simulink model "Final_EWASP_VC"  (R2022a)
settings: Solver=ode1  StartTime=0.0  StopTime=24*3600  FixedStep=10  RelTol=1e-3
values from neighbouring files (symbols this model uses):
  Aux_Threshold = 52    [Setup_Code_EWASP_VC.m]
  buildingAge = 2005    [Setup_Code_EWASP_VC.m]
  ceilingHeight = 2.4    [Setup_Code_EWASP_VC.m]
  conductiveHconnectMatrix = [ ... (first row only)    [Setup_Code_EWASP_VC.m]
  cRoofGreen = 100000    [Setup_Code_EWASP_VC.m]
  Defrost_After_Time = 30    [Setup_Code_EWASP_VC.m]
  DHWDemandProfile = occFreegainHotwaterElecTestPassiveOcc3(:,3)    [Setup_Code_EWASP_VC.m]
  Elec_Max = Elec_Max*(30/24.2)    [Setup_Code_EWASP_VC.m]
  Elec_Mid = Elec_Mid*(30/24.2)    [Setup_Code_EWASP_VC.m]
  Elec_Min = Elec_Min*(30/24.2)    [Setup_Code_EWASP_VC.m]
  ElecDemandProfile = occFreegainHotwaterElecTestPassiveOcc3(:,4)    [Setup_Code_EWASP_VC.m]
  ElecFixed = [Elec_Max(6,2) Elec_Max(6,4) Elec_Max(6,6) Elec_Max(6,7) ... (first row only)    [Setup_Code_EWASP_VC.m]
  floorOrCeilingArea = floorOrCeilingArea*1.15    [Setup_Code_EWASP_VC.m]
  forceCold = 0    [Setup_Code_EWASP_VC.m]
  freegain = occFreegainHotwaterElecTestPassiveOcc3(:,2)-max(occupancy)*25    [Setup_Code_EWASP_VC.m]
  furnitureModelOn = 1    [Setup_Code_EWASP_VC.m]
  Heat_Max = Heat_Max*(30/24.2)    [Setup_Code_EWASP_VC.m]
  Heat_Mid = Heat_Mid*(30/24.2)    [Setup_Code_EWASP_VC.m]
  Heat_Min = Heat_Min*(30/24.2)    [Setup_Code_EWASP_VC.m]
  HeatFixed = [Heat_Max(6,2) Heat_Max(6,4) Heat_Max(6,6) Heat_Max(6,7) ... (first row only)    [Setup_Code_EWASP_VC.m]
  HeatingOnProfile = repmat(HeatingOnProfile,365,1)    [Setup_Code_EWASP_VC.m]
  HEX_ReturnLowerLimit = 52.5    [Setup_Code_EWASP_VC.m]
  HEX_ReturnUpperLimit = 55    [Setup_Code_EWASP_VC.m]
  LeakMultiplier = 1+(2*(rand()-0.5)/10)    [Setup_Code_EWASP_VC.m]
  loopCap = 15    [Setup_Code_EWASP_VC.m]
  maxOcc = max(occupancyProfile)    [Setup_Code_EWASP_VC.m]
  NESW_wallArea = max(NESW_Lengths*ceilingHeight-NESW_Windows,0)    [Setup_Code_EWASP_VC.m]
  NESW_Windows = [ ... (first row only)    [Setup_Code_EWASP_VC.m]
  numRooms = roomCount    [Setup_Code_EWASP_VC.m]
  offsetDays = 0    [Setup_Code_EWASP_VC.m]
  pumpChoice = pumpChoices(MinIndex,1)    [Setup_Code_EWASP_VC.m]
  pumpRamp = 180    [Setup_Code_EWASP_VC.m]
  ReturnLowerLimit = 37.5    [Setup_Code_EWASP_VC.m]
  ReturnUpperLimit = 40    [Setup_Code_EWASP_VC.m]
  RoofIrradiance = Flat_NS_EW_RoofIrradiance(:,1)    [Setup_Code_EWASP_VC.m]
  roofStartTemp = ones(11,1)*20    [Setup_Code_EWASP_VC.m]
  rooftype = 0    [Setup_Code_EWASP_VC.m]
  RoomDataMatrix = [zeros(1,12);ones(1,12)*wallDensity;zeros(1,12);ones(1,12)*wallU;ones(1,12)*windowU;ones(1,12)*floorU;ones(1,12)*ceilingU;zeros(1,12);windowArea, 0;floorOrCeilingArea;zeros(1,12);floorOrCeilingArea*ceilingHeight]    [Setup_Code_EWASP_VC.m]
  roomVol = roomVol*1.15    [Setup_Code_EWASP_VC.m]
  slabStartTemp = (GroundTempTimeSeries(offsetDays*1440+1,1)+thermostatSetting)/2    [Setup_Code_EWASP_VC.m]
  SlackRequest = zeros(1440,1)    [Setup_Code_EWASP_VC.m]
  SolarThermalExists = 0    [Setup_Code_EWASP_VC.m]
  SourceFixed = HeatFixed-ElecFixed    [Setup_Code_EWASP_VC.m]
  StateSeries = StateSeriesGenerator(22,7,1)    [Setup_Code_EWASP_VC.m]
  Tank_Lower_Temp = 49.5    [Setup_Code_EWASP_VC.m]
  Tank_Upper_Temp = 52    [Setup_Code_EWASP_VC.m]
  Tank_Volume_m3 = 0.15    [Setup_Code_EWASP_VC.m]
  TankHeatHour = randi([1 5])-1    [Setup_Code_EWASP_VC.m]
  thermostatSetting = 20.0    (= 20)    [Setup_Code_EWASP_VC.m]
  upDown = [0;0;0;0;1;1;1;1;1;1;1]    [Setup_Code_EWASP_VC.m]
  variableASHP = 1    [Setup_Code_EWASP_VC.m]
  wallStartTempExt = thermostatSetting*(0.266+0.00215*outdoorStartTemp+0.018*wallU+0.00113*outdoorStartTemp*wallU+0.0068*wallU^2)    [Setup_Code_EWASP_VC.m]
undefined symbols (not defined in the file or in its folder): a, ceilingU, condUDMatrix, convUDMatrix, deltaPEXPANDED_E, deltaPEXPANDED_E2, deltaPEXPANDED_N, deltaPEXPANDED_N2, deltaPEXPANDED_S, deltaPEXPANDED_S2, deltaPEXPANDED_W, deltaPEXPANDED_W2, DesiredDHWTemp, DesiredFlowTempVsInOutDeltaTemp, DiffuseHorizontal, DiscIntNeverNeededParam, DNI, dwnAndConcrete, DWORK_A_HX, DWORK_CHK_FLU, DWORK_CP_NODE, DWORK_DH, DWORK_FLUID, DWORK_HCON, DWORK_LOSS, DWORK_MDOTDOWN, DWORK_MDOTIN, DWORK_MDOTUP, DWORK_MIX, DWORK_PRESS, DWORK_QDOTIN, DWORK_RHO_NODE, DWORK_TIN, DWORK_TS_OLD, DWORK_V_NODE, GroundTempTimeSeries, HCM, HCM2, HCM_closed, HCM_closed2, intermediateU, IsTop, massFlowMatrix, neighbourMatrix, numericalRoomUse, RadiatorMatrix, room2roomflowmatrix_E, room2roomflowmatrix_E2, room2roomflowmatrix_N, room2roomflowmatrix_N2, room2roomflowmatrix_S, room2roomflowmatrix_S2, room2roomflowmatrix_W, room2roomflowmatrix_W2, StateAirInEXPANDED_E, StateAirInEXPANDED_E2, StateAirInEXPANDED_N, StateAirInEXPANDED_N2, StateAirInEXPANDED_S, StateAirInEXPANDED_S2 ... (+23)
libraries: simulink x6, dspsigops x4, dspmtrx3 x4, carnot x3, spsEdgeDetectorLib x2, dspstat3 x2, powerlib_meascontrol x1, simulink_extras x1
(part 25 of 27)

== matlab function Final_EWASP_VC/Subsystem_Room2/Kitchen/furniture/MATLAB Function ==
  data: roomArea input; woodPlasticHeatTransfertoroom output; roomtype input; roomTemp input; TemperatureWoodPlastic input; TemperatureSoft input; deltaTWoodPlasticMean output; softHeatTransfertoroom output; deltaTsoftMean output
function [woodPlasticHeatTransfertoroom,deltaTWoodPlasticMean,softHeatTransfertoroom,deltaTsoftMean]=FurnitureTransfer(roomArea,roomtype,roomTemp,TemperatureWoodPlastic,TemperatureSoft)

excessMeanWoodPlastic=TemperatureWoodPlastic-roomTemp;
excessMeanSoft=TemperatureSoft-roomTemp;

if roomtype==1
    
%carpetMass=roomArea*2.041;% 2.041kg/m2 based on  https://thecarpetstop.co.uk/buying-guides/#:~:text=These%20are%20given%20in%20ounces,commonly%20a%20more%20luxurious%20carpet.  
%underlayMass=roomArea*2.7;% 2.7kg/m2 based on https://www.carpet-underlay-shop.co.uk/products/duralay-durafit-650-15-07m2-from-5-74-per-m2
CurtainMass=15;
Sofafabricmass=10;% based on 2lb/ft^3 and 2 sofas - 3 seater and 2 seater https://furnitureblog.simplicitysofas.com/blog/what-is-the-difference-between-a-sofa-cushions-foam-density-and-firmness/ 
matressMass=0; %no beds
duvetandSheetsMass=0; %no beds

SoftMass=CurtainMass+Sofafabricmass;
woodPlasticMass=roomArea*20-SoftMass;

elseif roomtype ==2

%carpetMass=roomArea*2.041;% 2.041kg/m2 based on  https://thecarpetstop.co.uk/buying-guides/#:~:text=These%20are%20given%20in%20ounces,commonly%20a%20more%20luxurious%20carpet.  
%underlayMass=roomArea*2.7;% 2.7kg/m2 based on https://www.carpet-underlay-shop.co.uk/products/duralay-durafit-650-15-07m2-from-5-74-per-m2
CurtainMass=15;
matressMass=40; %https://democracy.york.gov.uk/documents/s2116/Annex%20C%20REcycling%20Report%20frnweights2005.pdf
duvetandSheetsMass=5; %5kg based on %https://inthewash.co.uk/washing-machines/can-you-wash-a-king-size-duvet-in-an-8-9-10-kg-washing-machine/#:~:text=A%20king%20size%20duvet%20will,able%20to%20cope%20with%20them.
Sofafabricmass=0; %no sofa

SoftMass=CurtainMass+matressMass+duvetandSheetsMass;


woodPlasticMass=roomArea*30-SoftMass;
woodPlasticMass=roomArea*30-SoftMass;

else %room is other e.g. kitchen - assume heavily furnished, and majority wood or plastic
    
CurtainMass=0; %
matressMass=0; %
duvetandSheetsMass=0; %
Sofafabricmass=0; %no sofa

SoftMass=0;

woodPlasticMass=roomArea*35-SoftMass;
woodPlasticMass=roomArea*35-SoftMass;    
    
end





softDensityA=60;
softDensityB=80;
softThicknessA=0.15; %represents thicker furnishings (sofa foam etc.)
softThicknessB=0.01; %Represents thinner funishings (e.g. carpet)

SoftMassA=duvetandSheetsMass+Sofafabricmass+matressMass;
SoftMassB=CurtainMass;

SoftVolumeA=SoftMassA/softDensityA;
SoftVolumeB=SoftMassA/softDensityB;

approxSoftA_SA=(SoftVolumeA/softThicknessA);%no 2* here due to one surface usually being obscured
approxSoftB_SA=(SoftVolumeB/softThicknessB);%as above

Softradius=3*((SoftVolumeA+SoftVolumeB)/(approxSoftA_SA+approxSoftB_SA));
SoftbiotNumber=(10/0.03)*((SoftVolumeA+SoftVolumeB)/(approxSoftA_SA+approxSoftB_SA));% appropriate for typical soft furnishings with conductivity 0.03 w/mK and convective transfer coefficient 10 W/k m2 
SoftFBI=1/(0.282*SoftbiotNumber+0.944);
excessSurfSoft=SoftFBI*excessMeanSoft;
softHeatTransfertoroom=excessSurfSoft*10*(approxSoftA_SA+approxSoftB_SA);
deltaTsoftMean=-softHeatTransfertoroom/(softDensityA*SoftVolumeA*1400+softDensityB*SoftVolumeB*1400);

if isnan(deltaTsoftMean)==1
deltaTsoftMean=0;
else
end
    
woodPlasticDensity=800; %600kg/m^3 as of Influence of internal thermal mass on the indoor thermal dynamics and integration of phase change materials in furniture for building energy storage: A review
woodPlasticThickness=0.018; %0.018m typical as of as of Influence of internal thermal mass on the indoor thermal dynamics and integration of phase change materials in furniture for building energy storage: A review
woodPlasticVolume=woodPlasticMass/woodPlasticDensity;
approxWoodPlasticSA=(woodPlasticVolume/woodPlasticThickness); %a rough surface area calculation for the wooden elements

radius=3*woodPlasticVolume/approxWoodPlasticSA;
biotNumber=(10/0.2)*(woodPlasticVolume/approxWoodPlasticSA);% appropriate for typical wood with conductivity 0.2 w/mK and convective transfer coefficient 10 W/k m2 
FBI=1/(0.282*biotNumber+0.944);
excessSurfWoodPlastic=FBI*excessMeanWoodPlastic;
woodPlasticHeatTransfertoroom=excessSurfWoodPlastic*10*approxWoodPlasticSA;
deltaTWoodPlasticMean=-woodPlasticHeatTransfertoroom/(800*woodPlasticVolume*1700);% heat capacity of wodd and plastic is assumer 1700 J/Kg, they are very close in capacity anyway (1.76 wood, 1.67 plastic)

deltaTWoodPlasticMean(isnan(deltaTWoodPlasticMean))=0;

softHeatTransfertoroom(isnan(softHeatTransfertoroom))=0;

%end

== matlab function Final_EWASP_VC/Subsystem_Room3/Utility/furniture/MATLAB Function ==
  data: roomArea input; woodPlasticHeatTransfertoroom output; roomtype input; roomTemp input; TemperatureWoodPlastic input; TemperatureSoft input; deltaTWoodPlasticMean output; softHeatTransfertoroom output; deltaTsoftMean output
function [woodPlasticHeatTransfertoroom,deltaTWoodPlasticMean,softHeatTransfertoroom,deltaTsoftMean]=FurnitureTransfer(roomArea,roomtype,roomTemp,TemperatureWoodPlastic,TemperatureSoft)

excessMeanWoodPlastic=TemperatureWoodPlastic-roomTemp;
excessMeanSoft=TemperatureSoft-roomTemp;

if roomtype==1
    
%carpetMass=roomArea*2.041;% 2.041kg/m2 based on  https://thecarpetstop.co.uk/buying-guides/#:~:text=These%20are%20given%20in%20ounces,commonly%20a%20more%20luxurious%20carpet.  
%underlayMass=roomArea*2.7;% 2.7kg/m2 based on https://www.carpet-underlay-shop.co.uk/products/duralay-durafit-650-15-07m2-from-5-74-per-m2
CurtainMass=15;
Sofafabricmass=10;% based on 2lb/ft^3 and 2 sofas - 3 seater and 2 seater https://furnitureblog.simplicitysofas.com/blog/what-is-the-difference-between-a-sofa-cushions-foam-density-and-firmness/ 
matressMass=0; %no beds
duvetandSheetsMass=0; %no beds

SoftMass=CurtainMass+Sofafabricmass;
woodPlasticMass=roomArea*20-SoftMass;

elseif roomtype ==2

%carpetMass=roomArea*2.041;% 2.041kg/m2 based on  https://thecarpetstop.co.uk/buying-guides/#:~:text=These%20are%20given%20in%20ounces,commonly%20a%20more%20luxurious%20carpet.  
%underlayMass=roomArea*2.7;% 2.7kg/m2 based on https://www.carpet-underlay-shop.co.uk/products/duralay-durafit-650-15-07m2-from-5-74-per-m2
CurtainMass=15;
matressMass=40; %https://democracy.york.gov.uk/documents/s2116/Annex%20C%20REcycling%20Report%20frnweights2005.pdf
duvetandSheetsMass=5; %5kg based on %https://inthewash.co.uk/washing-machines/can-you-wash-a-king-size-duvet-in-an-8-9-10-kg-washing-machine/#:~:text=A%20king%20size%20duvet%20will,able%20to%20cope%20with%20them.
Sofafabricmass=0; %no sofa

SoftMass=CurtainMass+matressMass+duvetandSheetsMass;


woodPlasticMass=roomArea*30-SoftMass;
woodPlasticMass=roomArea*30-SoftMass;

else %room is other e.g. kitchen - assume heavily furnished, and majority wood or plastic
    
CurtainMass=0; %
matressMass=0; %
duvetandSheetsMass=0; %
Sofafabricmass=0; %no sofa

SoftMass=0;

woodPlasticMass=roomArea*35-SoftMass;
woodPlasticMass=roomArea*35-SoftMass;    
    
end





softDensityA=60;
softDensityB=80;
softThicknessA=0.15; %represents thicker furnishings (sofa foam etc.)
softThicknessB=0.01; %Represents thinner funishings (e.g. carpet)

SoftMassA=duvetandSheetsMass+Sofafabricmass+matressMass;
SoftMassB=CurtainMass;

SoftVolumeA=SoftMassA/softDensityA;
SoftVolumeB=SoftMassA/softDensityB;

approxSoftA_SA=(SoftVolumeA/softThicknessA);%no 2* here due to one surface usually being obscured
approxSoftB_SA=(SoftVolumeB/softThicknessB);%as above

Softradius=3*((SoftVolumeA+SoftVolumeB)/(approxSoftA_SA+approxSoftB_SA));
SoftbiotNumber=(10/0.03)*((SoftVolumeA+SoftVolumeB)/(approxSoftA_SA+approxSoftB_SA));% appropriate for typical soft furnishings with conductivity 0.03 w/mK and convective transfer coefficient 10 W/k m2 
SoftFBI=1/(0.282*SoftbiotNumber+0.944);
excessSurfSoft=SoftFBI*excessMeanSoft;
softHeatTransfertoroom=excessSurfSoft*10*(approxSoftA_SA+approxSoftB_SA);
deltaTsoftMean=-softHeatTransfertoroom/(softDensityA*SoftVolumeA*1400+softDensityB*SoftVolumeB*1400);

if isnan(deltaTsoftMean)==1
deltaTsoftMean=0;
else
end
    
woodPlasticDensity=800; %600kg/m^3 as of Influence of internal thermal mass on the indoor thermal dynamics and integration of phase change materials in furniture for building energy storage: A review
woodPlasticThickness=0.018; %0.018m typical as of as of Influence of internal thermal mass on the indoor thermal dynamics and integration of phase change materials in furniture for building energy storage: A review
woodPlasticVolume=woodPlasticMass/woodPlasticDensity;
approxWoodPlasticSA=(woodPlasticVolume/woodPlasticThickness); %a rough surface area calculation for the wooden elements

radius=3*woodPlasticVolume/approxWoodPlasticSA;
biotNumber=(10/0.2)*(woodPlasticVolume/approxWoodPlasticSA);% appropriate for typical wood with conductivity 0.2 w/mK and convective transfer coefficient 10 W/k m2 
FBI=1/(0.282*biotNumber+0.944);
excessSurfWoodPlastic=FBI*excessMeanWoodPlastic;
woodPlasticHeatTransfertoroom=excessSurfWoodPlastic*10*approxWoodPlasticSA;
deltaTWoodPlasticMean=-woodPlasticHeatTransfertoroom/(800*woodPlasticVolume*1700);% heat capacity of wodd and plastic is assumer 1700 J/Kg, they are very close in capacity anyway (1.76 wood, 1.67 plastic)

deltaTWoodPlasticMean(isnan(deltaTWoodPlasticMean))=0;

softHeatTransfertoroom(isnan(softHeatTransfertoroom))=0;

%end

== matlab function Final_EWASP_VC/Subsystem_Room4/Hall/furniture/MATLAB Function ==
  data: roomArea input; woodPlasticHeatTransfertoroom output; roomtype input; roomTemp input; TemperatureWoodPlastic input; TemperatureSoft input; deltaTWoodPlasticMean output; softHeatTransfertoroom output; deltaTsoftMean output
function [woodPlasticHeatTransfertoroom,deltaTWoodPlasticMean,softHeatTransfertoroom,deltaTsoftMean]=FurnitureTransfer(roomArea,roomtype,roomTemp,TemperatureWoodPlastic,TemperatureSoft)

excessMeanWoodPlastic=TemperatureWoodPlastic-roomTemp;
excessMeanSoft=TemperatureSoft-roomTemp;

if roomtype==1
    
%carpetMass=roomArea*2.041;% 2.041kg/m2 based on  https://thecarpetstop.co.uk/buying-guides/#:~:text=These%20are%20given%20in%20ounces,commonly%20a%20more%20luxurious%20carpet.  
%underlayMass=roomArea*2.7;% 2.7kg/m2 based on https://www.carpet-underlay-shop.co.uk/products/duralay-durafit-650-15-07m2-from-5-74-per-m2
CurtainMass=15;
Sofafabricmass=10;% based on 2lb/ft^3 and 2 sofas - 3 seater and 2 seater https://furnitureblog.simplicitysofas.com/blog/what-is-the-difference-between-a-sofa-cushions-foam-density-and-firmness/ 
matressMass=0; %no beds
duvetandSheetsMass=0; %no beds

SoftMass=CurtainMass+Sofafabricmass;
woodPlasticMass=roomArea*20-SoftMass;

elseif roomtype ==2

%carpetMass=roomArea*2.041;% 2.041kg/m2 based on  https://thecarpetstop.co.uk/buying-guides/#:~:text=These%20are%20given%20in%20ounces,commonly%20a%20more%20luxurious%20carpet.  
%underlayMass=roomArea*2.7;% 2.7kg/m2 based on https://www.carpet-underlay-shop.co.uk/products/duralay-durafit-650-15-07m2-from-5-74-per-m2
CurtainMass=15;
matressMass=40; %https://democracy.york.gov.uk/documents/s2116/Annex%20C%20REcycling%20Report%20frnweights2005.pdf
duvetandSheetsMass=5; %5kg based on %https://inthewash.co.uk/washing-machines/can-you-wash-a-king-size-duvet-in-an-8-9-10-kg-washing-machine/#:~:text=A%20king%20size%20duvet%20will,able%20to%20cope%20with%20them.
Sofafabricmass=0; %no sofa

SoftMass=CurtainMass+matressMass+duvetandSheetsMass;


woodPlasticMass=roomArea*30-SoftMass;
woodPlasticMass=roomArea*30-SoftMass;

else %room is other e.g. kitchen - assume heavily furnished, and majority wood or plastic
    
CurtainMass=0; %
matressMass=0; %
duvetandSheetsMass=0; %
Sofafabricmass=0; %no sofa

SoftMass=0;

woodPlasticMass=roomArea*35-SoftMass;
woodPlasticMass=roomArea*35-SoftMass;    
    
end





softDensityA=60;
softDensityB=80;
softThicknessA=0.15; %represents thicker furnishings (sofa foam etc.)
softThicknessB=0.01; %Represents thinner funishings (e.g. carpet)

SoftMassA=duvetandSheetsMass+Sofafabricmass+matressMass;
SoftMassB=CurtainMass;

SoftVolumeA=SoftMassA/softDensityA;
SoftVolumeB=SoftMassA/softDensityB;

approxSoftA_SA=(SoftVolumeA/softThicknessA);%no 2* here due to one surface usually being obscured
approxSoftB_SA=(SoftVolumeB/softThicknessB);%as above

Softradius=3*((SoftVolumeA+SoftVolumeB)/(approxSoftA_SA+approxSoftB_SA));
SoftbiotNumber=(10/0.03)*((SoftVolumeA+SoftVolumeB)/(approxSoftA_SA+approxSoftB_SA));% appropriate for typical soft furnishings with conductivity 0.03 w/mK and convective transfer coefficient 10 W/k m2 
SoftFBI=1/(0.282*SoftbiotNumber+0.944);
excessSurfSoft=SoftFBI*excessMeanSoft;
softHeatTransfertoroom=excessSurfSoft*10*(approxSoftA_SA+approxSoftB_SA);
deltaTsoftMean=-softHeatTransfertoroom/(softDensityA*SoftVolumeA*1400+softDensityB*SoftVolumeB*1400);

if isnan(deltaTsoftMean)==1
deltaTsoftMean=0;
else
end
    
woodPlasticDensity=800; %600kg/m^3 as of Influence of internal thermal mass on the indoor thermal dynamics and integration of phase change materials in furniture for building energy storage: A review
woodPlasticThickness=0.018; %0.018m typical as of as of Influence of internal thermal mass on the indoor thermal dynamics and integration of phase change materials in furniture for building energy storage: A review
woodPlasticVolume=woodPlasticMass/woodPlasticDensity;
approxWoodPlasticSA=(woodPlasticVolume/woodPlasticThickness); %a rough surface area calculation for the wooden elements

radius=3*woodPlasticVolume/approxWoodPlasticSA;
biotNumber=(10/0.2)*(woodPlasticVolume/approxWoodPlasticSA);% appropriate for typical wood with conductivity 0.2 w/mK and convective transfer coefficient 10 W/k m2 
FBI=1/(0.282*biotNumber+0.944);
excessSurfWoodPlastic=FBI*excessMeanWoodPlastic;
woodPlasticHeatTransfertoroom=excessSurfWoodPlastic*10*approxWoodPlasticSA;
deltaTWoodPlasticMean=-woodPlasticHeatTransfertoroom/(800*woodPlasticVolume*1700);% heat capacity of wodd and plastic is assumer 1700 J/Kg, they are very close in capacity anyway (1.76 wood, 1.67 plastic)

deltaTWoodPlasticMean(isnan(deltaTWoodPlasticMean))=0;

softHeatTransfertoroom(isnan(softHeatTransfertoroom))=0;

%end

== matlab function Final_EWASP_VC/Subsystem_Room5/Landing/furniture/MATLAB Function ==
  data: roomArea input; woodPlasticHeatTransfertoroom output; roomtype input; roomTemp input; TemperatureWoodPlastic input; TemperatureSoft input; deltaTWoodPlasticMean output; softHeatTransfertoroom output; deltaTsoftMean output
function [woodPlasticHeatTransfertoroom,deltaTWoodPlasticMean,softHeatTransfertoroom,deltaTsoftMean]=FurnitureTransfer(roomArea,roomtype,roomTemp,TemperatureWoodPlastic,TemperatureSoft)

excessMeanWoodPlastic=TemperatureWoodPlastic-roomTemp;
excessMeanSoft=TemperatureSoft-roomTemp;

if roomtype==1
    
%carpetMass=roomArea*2.041;% 2.041kg/m2 based on  https://thecarpetstop.co.uk/buying-guides/#:~:text=These%20are%20given%20in%20ounces,commonly%20a%20more%20luxurious%20carpet.  
%underlayMass=roomArea*2.7;% 2.7kg/m2 based on https://www.carpet-underlay-shop.co.uk/products/duralay-durafit-650-15-07m2-from-5-74-per-m2
CurtainMass=15;
Sofafabricmass=10;% based on 2lb/ft^3 and 2 sofas - 3 seater and 2 seater https://furnitureblog.simplicitysofas.com/blog/what-is-the-difference-between-a-sofa-cushions-foam-density-and-firmness/ 
matressMass=0; %no beds
duvetandSheetsMass=0; %no beds

SoftMass=CurtainMass+Sofafabricmass;
woodPlasticMass=roomArea*20-SoftMass;

elseif roomtype ==2

%carpetMass=roomArea*2.041;% 2.041kg/m2 based on  https://thecarpetstop.co.uk/buying-guides/#:~:text=These%20are%20given%20in%20ounces,commonly%20a%20more%20luxurious%20carpet.  
%underlayMass=roomArea*2.7;% 2.7kg/m2 based on https://www.carpet-underlay-shop.co.uk/products/duralay-durafit-650-15-07m2-from-5-74-per-m2
CurtainMass=15;
matressMass=40; %https://democracy.york.gov.uk/documents/s2116/Annex%20C%20REcycling%20Report%20frnweights2005.pdf
duvetandSheetsMass=5; %5kg based on %https://inthewash.co.uk/washing-machines/can-you-wash-a-king-size-duvet-in-an-8-9-10-kg-washing-machine/#:~:text=A%20king%20size%20duvet%20will,able%20to%20cope%20with%20them.
Sofafabricmass=0; %no sofa

SoftMass=CurtainMass+matressMass+duvetandSheetsMass;


woodPlasticMass=roomArea*30-SoftMass;
woodPlasticMass=roomArea*30-SoftMass;

else %room is other e.g. kitchen - assume heavily furnished, and majority wood or plastic
    
CurtainMass=0; %
matressMass=0; %
duvetandSheetsMass=0; %
Sofafabricmass=0; %no sofa

SoftMass=0;

woodPlasticMass=roomArea*35-SoftMass;
woodPlasticMass=roomArea*35-SoftMass;    
    
end





softDensityA=60;
softDensityB=80;
softThicknessA=0.15; %represents thicker furnishings (sofa foam etc.)
softThicknessB=0.01; %Represents thinner funishings (e.g. carpet)

SoftMassA=duvetandSheetsMass+Sofafabricmass+matressMass;
SoftMassB=CurtainMass;

SoftVolumeA=SoftMassA/softDensityA;
SoftVolumeB=SoftMassA/softDensityB;

approxSoftA_SA=(SoftVolumeA/softThicknessA);%no 2* here due to one surface usually being obscured
approxSoftB_SA=(SoftVolumeB/softThicknessB);%as above

Softradius=3*((SoftVolumeA+SoftVolumeB)/(approxSoftA_SA+approxSoftB_SA));
SoftbiotNumber=(10/0.03)*((SoftVolumeA+SoftVolumeB)/(approxSoftA_SA+approxSoftB_SA));% appropriate for typical soft furnishings with conductivity 0.03 w/mK and convective transfer coefficient 10 W/k m2 
SoftFBI=1/(0.282*SoftbiotNumber+0.944);
excessSurfSoft=SoftFBI*excessMeanSoft;
softHeatTransfertoroom=excessSurfSoft*10*(approxSoftA_SA+approxSoftB_SA);
deltaTsoftMean=-softHeatTransfertoroom/(softDensityA*SoftVolumeA*1400+softDensityB*SoftVolumeB*1400);

if isnan(deltaTsoftMean)==1
deltaTsoftMean=0;
else
end
    
woodPlasticDensity=800; %600kg/m^3 as of Influence of internal thermal mass on the indoor thermal dynamics and integration of phase change materials in furniture for building energy storage: A review
woodPlasticThickness=0.018; %0.018m typical as of as of Influence of internal thermal mass on the indoor thermal dynamics and integration of phase change materials in furniture for building energy storage: A review
woodPlasticVolume=woodPlasticMass/woodPlasticDensity;
approxWoodPlasticSA=(woodPlasticVolume/woodPlasticThickness); %a rough surface area calculation for the wooden elements

radius=3*woodPlasticVolume/approxWoodPlasticSA;
biotNumber=(10/0.2)*(woodPlasticVolume/approxWoodPlasticSA);% appropriate for typical wood with conductivity 0.2 w/mK and convective transfer coefficient 10 W/k m2 
FBI=1/(0.282*biotNumber+0.944);
excessSurfWoodPlastic=FBI*excessMeanWoodPlastic;
woodPlasticHeatTransfertoroom=excessSurfWoodPlastic*10*approxWoodPlasticSA;
deltaTWoodPlasticMean=-woodPlasticHeatTransfertoroom/(800*woodPlasticVolume*1700);% heat capacity of wodd and plastic is assumer 1700 J/Kg, they are very close in capacity anyway (1.76 wood, 1.67 plastic)

deltaTWoodPlasticMean(isnan(deltaTWoodPlasticMean))=0;

softHeatTransfertoroom(isnan(softHeatTransfertoroom))=0;

%end

== matlab function Final_EWASP_VC/Subsystem_Room4/Hall/Subsystem1/MATLAB Function1 ==
  data: PU_AreaIrradianceTotal output; angleSeries input; NEWS_Irradiance output; DNISeries input; DiffSeries input; Time input; offsetDays input; SurfaceAlbedo input; NESW_wallArea input; roomNumber input; c_OutPU input; deltaTexternalNEWS output
function [PU_AreaIrradianceTotal, NEWS_Irradiance,deltaTexternalNEWS] = SolarSeriesToExtWallGains(angleSeries,DNISeries,DiffSeries,Time,offsetDays,SurfaceAlbedo,NESW_wallArea,roomNumber,c_OutPU)

%deltaTexternalNEWS=zeros(1,4);

Angle_NEWS=angleSeries(ceil((offsetDays*1440)+Time/60+0.00001),1:4);
DNI=DNISeries(ceil((offsetDays*1440)+Time/60+0.00001),1);

PU_AreaDiff=DiffSeries(ceil((offsetDays*1440)+Time/60+0.00001),1)/2;%extracts correct Diff for the timestep, factor of 1/2 corrects for 90 degree walls (so only half Diff irradiance can be utilised)
PU_AreaDNI=cos(deg2rad(Angle_NEWS))*DNI;
NEWS_wallArea=NESW_wallArea;
NEWS_wallArea([3 4],:)=NEWS_wallArea([4 3],:);

RoomWallAreas_NEWS=NEWS_wallArea(:,roomNumber)';
PU_AreaIrradianceTotal=(PU_AreaDNI+PU_AreaDiff)*(1-SurfaceAlbedo);

NEWS_Irradiance=RoomWallAreas_NEWS.*PU_AreaIrradianceTotal;
deltaTexternalNEWS=NEWS_Irradiance./(c_OutPU*RoomWallAreas_NEWS);

for i=1:4
   
    if RoomWallAreas_NEWS(1,i)==0
        deltaTexternalNEWS(1,i)=0;
    else
        
    end
    
end

== matlab function Final_EWASP_VC/Subsystem_Room6/Bedroom1/furniture/MATLAB Function ==
  data: roomArea input; woodPlasticHeatTransfertoroom output; roomtype input; roomTemp input; TemperatureWoodPlastic input; TemperatureSoft input; deltaTWoodPlasticMean output; softHeatTransfertoroom output; deltaTsoftMean output
function [woodPlasticHeatTransfertoroom,deltaTWoodPlasticMean,softHeatTransfertoroom,deltaTsoftMean]=FurnitureTransfer(roomArea,roomtype,roomTemp,TemperatureWoodPlastic,TemperatureSoft)

excessMeanWoodPlastic=TemperatureWoodPlastic-roomTemp;
excessMeanSoft=TemperatureSoft-roomTemp;

if roomtype==1
    
%carpetMass=roomArea*2.041;% 2.041kg/m2 based on  https://thecarpetstop.co.uk/buying-guides/#:~:text=These%20are%20given%20in%20ounces,commonly%20a%20more%20luxurious%20carpet.  
%underlayMass=roomArea*2.7;% 2.7kg/m2 based on https://www.carpet-underlay-shop.co.uk/products/duralay-durafit-650-15-07m2-from-5-74-per-m2
CurtainMass=15;
Sofafabricmass=10;% based on 2lb/ft^3 and 2 sofas - 3 seater and 2 seater https://furnitureblog.simplicitysofas.com/blog/what-is-the-difference-between-a-sofa-cushions-foam-density-and-firmness/ 
matressMass=0; %no beds
duvetandSheetsMass=0; %no beds

SoftMass=CurtainMass+Sofafabricmass;
woodPlasticMass=roomArea*20-SoftMass;

elseif roomtype ==2

%carpetMass=roomArea*2.041;% 2.041kg/m2 based on  https://thecarpetstop.co.uk/buying-guides/#:~:text=These%20are%20given%20in%20ounces,commonly%20a%20more%20luxurious%20carpet.  
%underlayMass=roomArea*2.7;% 2.7kg/m2 based on https://www.carpet-underlay-shop.co.uk/products/duralay-durafit-650-15-07m2-from-5-74-per-m2
CurtainMass=15;
matressMass=40; %https://democracy.york.gov.uk/documents/s2116/Annex%20C%20REcycling%20Report%20frnweights2005.pdf
duvetandSheetsMass=5; %5kg based on %https://inthewash.co.uk/washing-machines/can-you-wash-a-king-size-duvet-in-an-8-9-10-kg-washing-machine/#:~:text=A%20king%20size%20duvet%20will,able%20to%20cope%20with%20them.
Sofafabricmass=0; %no sofa

SoftMass=CurtainMass+matressMass+duvetandSheetsMass;


woodPlasticMass=roomArea*30-SoftMass;
woodPlasticMass=roomArea*30-SoftMass;

else %room is other e.g. kitchen - assume heavily furnished, and majority wood or plastic
    
CurtainMass=0; %
matressMass=0; %
duvetandSheetsMass=0; %
Sofafabricmass=0; %no sofa

SoftMass=0;

woodPlasticMass=roomArea*35-SoftMass;
woodPlasticMass=roomArea*35-SoftMass;    
    
end





softDensityA=60;
softDensityB=80;
softThicknessA=0.15; %represents thicker furnishings (sofa foam etc.)
softThicknessB=0.01; %Represents thinner funishings (e.g. carpet)

SoftMassA=duvetandSheetsMass+Sofafabricmass+matressMass;
SoftMassB=CurtainMass;

SoftVolumeA=SoftMassA/softDensityA;
SoftVolumeB=SoftMassA/softDensityB;

approxSoftA_SA=(SoftVolumeA/softThicknessA);%no 2* here due to one surface usually being obscured
approxSoftB_SA=(SoftVolumeB/softThicknessB);%as above

Softradius=3*((SoftVolumeA+SoftVolumeB)/(approxSoftA_SA+approxSoftB_SA));
SoftbiotNumber=(10/0.03)*((SoftVolumeA+SoftVolumeB)/(approxSoftA_SA+approxSoftB_SA));% appropriate for typical soft furnishings with conductivity 0.03 w/mK and convective transfer coefficient 10 W/k m2 
SoftFBI=1/(0.282*SoftbiotNumber+0.944);
excessSurfSoft=SoftFBI*excessMeanSoft;
softHeatTransfertoroom=excessSurfSoft*10*(approxSoftA_SA+approxSoftB_SA);
deltaTsoftMean=-softHeatTransfertoroom/(softDensityA*SoftVolumeA*1400+softDensityB*SoftVolumeB*1400);

if isnan(deltaTsoftMean)==1
deltaTsoftMean=0;
else
end
    
woodPlasticDensity=800; %600kg/m^3 as of Influence of internal thermal mass on the indoor thermal dynamics and integration of phase change materials in furniture for building energy storage: A review
woodPlasticThickness=0.018; %0.018m typical as of as of Influence of internal thermal mass on the indoor thermal dynamics and integration of phase change materials in furniture for building energy storage: A review
woodPlasticVolume=woodPlasticMass/woodPlasticDensity;
approxWoodPlasticSA=(woodPlasticVolume/woodPlasticThickness); %a rough surface area calculation for the wooden elements

radius=3*woodPlasticVolume/approxWoodPlasticSA;
biotNumber=(10/0.2)*(woodPlasticVolume/approxWoodPlasticSA);% appropriate for typical wood with conductivity 0.2 w/mK and convective transfer coefficient 10 W/k m2 
FBI=1/(0.282*biotNumber+0.944);
excessSurfWoodPlastic=FBI*excessMeanWoodPlastic;
woodPlasticHeatTransfertoroom=excessSurfWoodPlastic*10*approxWoodPlasticSA;
deltaTWoodPlasticMean=-woodPlasticHeatTransfertoroom/(800*woodPlasticVolume*1700);% heat capacity of wodd and plastic is assumer 1700 J/Kg, they are very close in capacity anyway (1.76 wood, 1.67 plastic)

deltaTWoodPlasticMean(isnan(deltaTWoodPlasticMean))=0;

softHeatTransfertoroom(isnan(softHeatTransfertoroom))=0;

%end

== matlab function Final_EWASP_VC/Subsystem_Room7/Bedroom 2/furniture/MATLAB Function ==
  data: roomArea input; woodPlasticHeatTransfertoroom output; roomtype input; roomTemp input; TemperatureWoodPlastic input; TemperatureSoft input; deltaTWoodPlasticMean output; softHeatTransfertoroom output; deltaTsoftMean output
function [woodPlasticHeatTransfertoroom,deltaTWoodPlasticMean,softHeatTransfertoroom,deltaTsoftMean]=FurnitureTransfer(roomArea,roomtype,roomTemp,TemperatureWoodPlastic,TemperatureSoft)

excessMeanWoodPlastic=TemperatureWoodPlastic-roomTemp;
excessMeanSoft=TemperatureSoft-roomTemp;

if roomtype==1
    
%carpetMass=roomArea*2.041;% 2.041kg/m2 based on  https://thecarpetstop.co.uk/buying-guides/#:~:text=These%20are%20given%20in%20ounces,commonly%20a%20more%20luxurious%20carpet.  
%underlayMass=roomArea*2.7;% 2.7kg/m2 based on https://www.carpet-underlay-shop.co.uk/products/duralay-durafit-650-15-07m2-from-5-74-per-m2
CurtainMass=15;
Sofafabricmass=10;% based on 2lb/ft^3 and 2 sofas - 3 seater and 2 seater https://furnitureblog.simplicitysofas.com/blog/what-is-the-difference-between-a-sofa-cushions-foam-density-and-firmness/ 
matressMass=0; %no beds
duvetandSheetsMass=0; %no beds

SoftMass=CurtainMass+Sofafabricmass;
woodPlasticMass=roomArea*20-SoftMass;

elseif roomtype ==2

%carpetMass=roomArea*2.041;% 2.041kg/m2 based on  https://thecarpetstop.co.uk/buying-guides/#:~:text=These%20are%20given%20in%20ounces,commonly%20a%20more%20luxurious%20carpet.  
%underlayMass=roomArea*2.7;% 2.7kg/m2 based on https://www.carpet-underlay-shop.co.uk/products/duralay-durafit-650-15-07m2-from-5-74-per-m2
CurtainMass=15;
matressMass=40; %https://democracy.york.gov.uk/documents/s2116/Annex%20C%20REcycling%20Report%20frnweights2005.pdf
duvetandSheetsMass=5; %5kg based on %https://inthewash.co.uk/washing-machines/can-you-wash-a-king-size-duvet-in-an-8-9-10-kg-washing-machine/#:~:text=A%20king%20size%20duvet%20will,able%20to%20cope%20with%20them.
Sofafabricmass=0; %no sofa

SoftMass=CurtainMass+matressMass+duvetandSheetsMass;


woodPlasticMass=roomArea*30-SoftMass;
woodPlasticMass=roomArea*30-SoftMass;

else %room is other e.g. kitchen - assume heavily furnished, and majority wood or plastic
    
CurtainMass=0; %
matressMass=0; %
duvetandSheetsMass=0; %
Sofafabricmass=0; %no sofa

SoftMass=0;

woodPlasticMass=roomArea*35-SoftMass;
woodPlasticMass=roomArea*35-SoftMass;    
    
end





softDensityA=60;
softDensityB=80;
softThicknessA=0.15; %represents thicker furnishings (sofa foam etc.)
softThicknessB=0.01; %Represents thinner funishings (e.g. carpet)

SoftMassA=duvetandSheetsMass+Sofafabricmass+matressMass;
SoftMassB=CurtainMass;

SoftVolumeA=SoftMassA/softDensityA;
SoftVolumeB=SoftMassA/softDensityB;

approxSoftA_SA=(SoftVolumeA/softThicknessA);%no 2* here due to one surface usually being obscured
approxSoftB_SA=(SoftVolumeB/softThicknessB);%as above

Softradius=3*((SoftVolumeA+SoftVolumeB)/(approxSoftA_SA+approxSoftB_SA));
SoftbiotNumber=(10/0.03)*((SoftVolumeA+SoftVolumeB)/(approxSoftA_SA+approxSoftB_SA));% appropriate for typical soft furnishings with conductivity 0.03 w/mK and convective transfer coefficient 10 W/k m2 
SoftFBI=1/(0.282*SoftbiotNumber+0.944);
excessSurfSoft=SoftFBI*excessMeanSoft;
softHeatTransfertoroom=excessSurfSoft*10*(approxSoftA_SA+approxSoftB_SA);
deltaTsoftMean=-softHeatTransfertoroom/(softDensityA*SoftVolumeA*1400+softDensityB*SoftVolumeB*1400);

if isnan(deltaTsoftMean)==1
deltaTsoftMean=0;
else
end
    
woodPlasticDensity=800; %600kg/m^3 as of Influence of internal thermal mass on the indoor thermal dynamics and integration of phase change materials in furniture for building energy storage: A review
woodPlasticThickness=0.018; %0.018m typical as of as of Influence of internal thermal mass on the indoor thermal dynamics and integration of phase change materials in furniture for building energy storage: A review
woodPlasticVolume=woodPlasticMass/woodPlasticDensity;
approxWoodPlasticSA=(woodPlasticVolume/woodPlasticThickness); %a rough surface area calculation for the wooden elements

radius=3*woodPlasticVolume/approxWoodPlasticSA;
biotNumber=(10/0.2)*(woodPlasticVolume/approxWoodPlasticSA);% appropriate for typical wood with conductivity 0.2 w/mK and convective transfer coefficient 10 W/k m2 
FBI=1/(0.282*biotNumber+0.944);
excessSurfWoodPlastic=FBI*excessMeanWoodPlastic;
woodPlasticHeatTransfertoroom=excessSurfWoodPlastic*10*approxWoodPlasticSA;
deltaTWoodPlasticMean=-woodPlasticHeatTransfertoroom/(800*woodPlasticVolume*1700);% heat capacity of wodd and plastic is assumer 1700 J/Kg, they are very close in capacity anyway (1.76 wood, 1.67 plastic)

deltaTWoodPlasticMean(isnan(deltaTWoodPlasticMean))=0;

softHeatTransfertoroom(isnan(softHeatTransfertoroom))=0;

%end

== matlab function Final_EWASP_VC/Subsystem_Room8/Bedroom3/furniture/MATLAB Function ==
  data: roomArea input; woodPlasticHeatTransfertoroom output; roomtype input; roomTemp input; TemperatureWoodPlastic input; TemperatureSoft input; deltaTWoodPlasticMean output; softHeatTransfertoroom output; deltaTsoftMean output
function [woodPlasticHeatTransfertoroom,deltaTWoodPlasticMean,softHeatTransfertoroom,deltaTsoftMean]=FurnitureTransfer(roomArea,roomtype,roomTemp,TemperatureWoodPlastic,TemperatureSoft)

excessMeanWoodPlastic=TemperatureWoodPlastic-roomTemp;
excessMeanSoft=TemperatureSoft-roomTemp;

if roomtype==1
    
%carpetMass=roomArea*2.041;% 2.041kg/m2 based on  https://thecarpetstop.co.uk/buying-guides/#:~:text=These%20are%20given%20in%20ounces,commonly%20a%20more%20luxurious%20carpet.  
%underlayMass=roomArea*2.7;% 2.7kg/m2 based on https://www.carpet-underlay-shop.co.uk/products/duralay-durafit-650-15-07m2-from-5-74-per-m2
CurtainMass=15;
Sofafabricmass=10;% based on 2lb/ft^3 and 2 sofas - 3 seater and 2 seater https://furnitureblog.simplicitysofas.com/blog/what-is-the-difference-between-a-sofa-cushions-foam-density-and-firmness/ 
matressMass=0; %no beds
duvetandSheetsMass=0; %no beds

SoftMass=CurtainMass+Sofafabricmass;
woodPlasticMass=roomArea*20-SoftMass;

elseif roomtype ==2

%carpetMass=roomArea*2.041;% 2.041kg/m2 based on  https://thecarpetstop.co.uk/buying-guides/#:~:text=These%20are%20given%20in%20ounces,commonly%20a%20more%20luxurious%20carpet.  
%underlayMass=roomArea*2.7;% 2.7kg/m2 based on https://www.carpet-underlay-shop.co.uk/products/duralay-durafit-650-15-07m2-from-5-74-per-m2
CurtainMass=15;
matressMass=40; %https://democracy.york.gov.uk/documents/s2116/Annex%20C%20REcycling%20Report%20frnweights2005.pdf
duvetandSheetsMass=5; %5kg based on %https://inthewash.co.uk/washing-machines/can-you-wash-a-king-size-duvet-in-an-8-9-10-kg-washing-machine/#:~:text=A%20king%20size%20duvet%20will,able%20to%20cope%20with%20them.
Sofafabricmass=0; %no sofa

SoftMass=CurtainMass+matressMass+duvetandSheetsMass;


woodPlasticMass=roomArea*30-SoftMass;
woodPlasticMass=roomArea*30-SoftMass;

else %room is other e.g. kitchen - assume heavily furnished, and majority wood or plastic
    
CurtainMass=0; %
matressMass=0; %
duvetandSheetsMass=0; %
Sofafabricmass=0; %no sofa

SoftMass=0;

woodPlasticMass=roomArea*35-SoftMass;
woodPlasticMass=roomArea*35-SoftMass;    
    
end





softDensityA=60;
softDensityB=80;
softThicknessA=0.15; %represents thicker furnishings (sofa foam etc.)
softThicknessB=0.01; %Represents thinner funishings (e.g. carpet)

SoftMassA=duvetandSheetsMass+Sofafabricmass+matressMass;
SoftMassB=CurtainMass;

SoftVolumeA=SoftMassA/softDensityA;
SoftVolumeB=SoftMassA/softDensityB;

approxSoftA_SA=(SoftVolumeA/softThicknessA);%no 2* here due to one surface usually being obscured
approxSoftB_SA=(SoftVolumeB/softThicknessB);%as above

Softradius=3*((SoftVolumeA+SoftVolumeB)/(approxSoftA_SA+approxSoftB_SA));
SoftbiotNumber=(10/0.03)*((SoftVolumeA+SoftVolumeB)/(approxSoftA_SA+approxSoftB_SA));% appropriate for typical soft furnishings with conductivity 0.03 w/mK and convective transfer coefficient 10 W/k m2 
SoftFBI=1/(0.282*SoftbiotNumber+0.944);
excessSurfSoft=SoftFBI*excessMeanSoft;
softHeatTransfertoroom=excessSurfSoft*10*(approxSoftA_SA+approxSoftB_SA);
deltaTsoftMean=-softHeatTransfertoroom/(softDensityA*SoftVolumeA*1400+softDensityB*SoftVolumeB*1400);

if isnan(deltaTsoftMean)==1
deltaTsoftMean=0;
else
end
    
woodPlasticDensity=800; %600kg/m^3 as of Influence of internal thermal mass on the indoor thermal dynamics and integration of phase change materials in furniture for building energy storage: A review
woodPlasticThickness=0.018; %0.018m typical as of as of Influence of internal thermal mass on the indoor thermal dynamics and integration of phase change materials in furniture for building energy storage: A review
woodPlasticVolume=woodPlasticMass/woodPlasticDensity;
approxWoodPlasticSA=(woodPlasticVolume/woodPlasticThickness); %a rough surface area calculation for the wooden elements

radius=3*woodPlasticVolume/approxWoodPlasticSA;
biotNumber=(10/0.2)*(woodPlasticVolume/approxWoodPlasticSA);% appropriate for typical wood with conductivity 0.2 w/mK and convective transfer coefficient 10 W/k m2 
FBI=1/(0.282*biotNumber+0.944);
excessSurfWoodPlastic=FBI*excessMeanWoodPlastic;
woodPlasticHeatTransfertoroom=excessSurfWoodPlastic*10*approxWoodPlasticSA;
deltaTWoodPlasticMean=-woodPlasticHeatTransfertoroom/(800*woodPlasticVolume*1700);% heat capacity of wodd and plastic is assumer 1700 J/Kg, they are very close in capacity anyway (1.76 wood, 1.67 plastic)

deltaTWoodPlasticMean(isnan(deltaTWoodPlasticMean))=0;

softHeatTransfertoroom(isnan(softHeatTransfertoroom))=0;

%end

== matlab function Final_EWASP_VC/Subsystem_Room9/Bedroom4/furniture/MATLAB Function ==
  data: roomArea input; woodPlasticHeatTransfertoroom output; roomtype input; roomTemp input; TemperatureWoodPlastic input; TemperatureSoft input; deltaTWoodPlasticMean output; softHeatTransfertoroom output; deltaTsoftMean output
function [woodPlasticHeatTransfertoroom,deltaTWoodPlasticMean,softHeatTransfertoroom,deltaTsoftMean]=FurnitureTransfer(roomArea,roomtype,roomTemp,TemperatureWoodPlastic,TemperatureSoft)

excessMeanWoodPlastic=TemperatureWoodPlastic-roomTemp;
excessMeanSoft=TemperatureSoft-roomTemp;

if roomtype==1
    
%carpetMass=roomArea*2.041;% 2.041kg/m2 based on  https://thecarpetstop.co.uk/buying-guides/#:~:text=These%20are%20given%20in%20ounces,commonly%20a%20more%20luxurious%20carpet.  
%underlayMass=roomArea*2.7;% 2.7kg/m2 based on https://www.carpet-underlay-shop.co.uk/products/duralay-durafit-650-15-07m2-from-5-74-per-m2
CurtainMass=15;
Sofafabricmass=10;% based on 2lb/ft^3 and 2 sofas - 3 seater and 2 seater https://furnitureblog.simplicitysofas.com/blog/what-is-the-difference-between-a-sofa-cushions-foam-density-and-firmness/ 
matressMass=0; %no beds
duvetandSheetsMass=0; %no beds

SoftMass=CurtainMass+Sofafabricmass;
woodPlasticMass=roomArea*20-SoftMass;

elseif roomtype ==2

%carpetMass=roomArea*2.041;% 2.041kg/m2 based on  https://thecarpetstop.co.uk/buying-guides/#:~:text=These%20are%20given%20in%20ounces,commonly%20a%20more%20luxurious%20carpet.  
%underlayMass=roomArea*2.7;% 2.7kg/m2 based on https://www.carpet-underlay-shop.co.uk/products/duralay-durafit-650-15-07m2-from-5-74-per-m2
CurtainMass=15;
matressMass=40; %https://democracy.york.gov.uk/documents/s2116/Annex%20C%20REcycling%20Report%20frnweights2005.pdf
duvetandSheetsMass=5; %5kg based on %https://inthewash.co.uk/washing-machines/can-you-wash-a-king-size-duvet-in-an-8-9-10-kg-washing-machine/#:~:text=A%20king%20size%20duvet%20will,able%20to%20cope%20with%20them.
Sofafabricmass=0; %no sofa

SoftMass=CurtainMass+matressMass+duvetandSheetsMass;


woodPlasticMass=roomArea*30-SoftMass;
woodPlasticMass=roomArea*30-SoftMass;

else %room is other e.g. kitchen - assume heavily furnished, and majority wood or plastic
    
CurtainMass=0; %
matressMass=0; %
duvetandSheetsMass=0; %
Sofafabricmass=0; %no sofa

SoftMass=0;

woodPlasticMass=roomArea*35-SoftMass;
woodPlasticMass=roomArea*35-SoftMass;    
    
end





softDensityA=60;
softDensityB=80;
softThicknessA=0.15; %represents thicker furnishings (sofa foam etc.)
softThicknessB=0.01; %Represents thinner funishings (e.g. carpet)

SoftMassA=duvetandSheetsMass+Sofafabricmass+matressMass;
SoftMassB=CurtainMass;

SoftVolumeA=SoftMassA/softDensityA;
SoftVolumeB=SoftMassA/softDensityB;

approxSoftA_SA=(SoftVolumeA/softThicknessA);%no 2* here due to one surface usually being obscured
approxSoftB_SA=(SoftVolumeB/softThicknessB);%as above

Softradius=3*((SoftVolumeA+SoftVolumeB)/(approxSoftA_SA+approxSoftB_SA));
SoftbiotNumber=(10/0.03)*((SoftVolumeA+SoftVolumeB)/(approxSoftA_SA+approxSoftB_SA));% appropriate for typical soft furnishings with conductivity 0.03 w/mK and convective transfer coefficient 10 W/k m2 
SoftFBI=1/(0.282*SoftbiotNumber+0.944);
excessSurfSoft=SoftFBI*excessMeanSoft;
softHeatTransfertoroom=excessSurfSoft*10*(approxSoftA_SA+approxSoftB_SA);
deltaTsoftMean=-softHeatTransfertoroom/(softDensityA*SoftVolumeA*1400+softDensityB*SoftVolumeB*1400);

if isnan(deltaTsoftMean)==1
deltaTsoftMean=0;
else
end
    
woodPlasticDensity=800; %600kg/m^3 as of Influence of internal thermal mass on the indoor thermal dynamics and integration of phase change materials in furniture for building energy storage: A review
woodPlasticThickness=0.018; %0.018m typical as of as of Influence of internal thermal mass on the indoor thermal dynamics and integration of phase change materials in furniture for building energy storage: A review
woodPlasticVolume=woodPlasticMass/woodPlasticDensity;
approxWoodPlasticSA=(woodPlasticVolume/woodPlasticThickness); %a rough surface area calculation for the wooden elements

radius=3*woodPlasticVolume/approxWoodPlasticSA;
biotNumber=(10/0.2)*(woodPlasticVolume/approxWoodPlasticSA);% appropriate for typical wood with conductivity 0.2 w/mK and convective transfer coefficient 10 W/k m2 
FBI=1/(0.282*biotNumber+0.944);
excessSurfWoodPlastic=FBI*excessMeanWoodPlastic;
woodPlasticHeatTransfertoroom=excessSurfWoodPlastic*10*approxWoodPlasticSA;
deltaTWoodPlasticMean=-woodPlasticHeatTransfertoroom/(800*woodPlasticVolume*1700);% heat capacity of wodd and plastic is assumer 1700 J/Kg, they are very close in capacity anyway (1.76 wood, 1.67 plastic)

deltaTWoodPlasticMean(isnan(deltaTWoodPlasticMean))=0;

softHeatTransfertoroom(isnan(softHeatTransfertoroom))=0;

%end

== matlab function Final_EWASP_VC/Subsystem_Room10/En suite/furniture/MATLAB Function ==
  data: roomArea input; woodPlasticHeatTransfertoroom output; roomtype input; roomTemp input; TemperatureWoodPlastic input; TemperatureSoft input; deltaTWoodPlasticMean output; softHeatTransfertoroom output; deltaTsoftMean output
function [woodPlasticHeatTransfertoroom,deltaTWoodPlasticMean,softHeatTransfertoroom,deltaTsoftMean]=FurnitureTransfer(roomArea,roomtype,roomTemp,TemperatureWoodPlastic,TemperatureSoft)

excessMeanWoodPlastic=TemperatureWoodPlastic-roomTemp;
excessMeanSoft=TemperatureSoft-roomTemp;

if roomtype==1
    
%carpetMass=roomArea*2.041;% 2.041kg/m2 based on  https://thecarpetstop.co.uk/buying-guides/#:~:text=These%20are%20given%20in%20ounces,commonly%20a%20more%20luxurious%20carpet.  
%underlayMass=roomArea*2.7;% 2.7kg/m2 based on https://www.carpet-underlay-shop.co.uk/products/duralay-durafit-650-15-07m2-from-5-74-per-m2
CurtainMass=15;
Sofafabricmass=10;% based on 2lb/ft^3 and 2 sofas - 3 seater and 2 seater https://furnitureblog.simplicitysofas.com/blog/what-is-the-difference-between-a-sofa-cushions-foam-density-and-firmness/ 
matressMass=0; %no beds
duvetandSheetsMass=0; %no beds

SoftMass=CurtainMass+Sofafabricmass;
woodPlasticMass=roomArea*20-SoftMass;

elseif roomtype ==2

%carpetMass=roomArea*2.041;% 2.041kg/m2 based on  https://thecarpetstop.co.uk/buying-guides/#:~:text=These%20are%20given%20in%20ounces,commonly%20a%20more%20luxurious%20carpet.  
%underlayMass=roomArea*2.7;% 2.7kg/m2 based on https://www.carpet-underlay-shop.co.uk/products/duralay-durafit-650-15-07m2-from-5-74-per-m2
CurtainMass=15;
matressMass=40; %https://democracy.york.gov.uk/documents/s2116/Annex%20C%20REcycling%20Report%20frnweights2005.pdf
duvetandSheetsMass=5; %5kg based on %https://inthewash.co.uk/washing-machines/can-you-wash-a-king-size-duvet-in-an-8-9-10-kg-washing-machine/#:~:text=A%20king%20size%20duvet%20will,able%20to%20cope%20with%20them.
Sofafabricmass=0; %no sofa

SoftMass=CurtainMass+matressMass+duvetandSheetsMass;


woodPlasticMass=roomArea*30-SoftMass;
woodPlasticMass=roomArea*30-SoftMass;

else %room is other e.g. kitchen - assume heavily furnished, and majority wood or plastic
    
CurtainMass=0; %
matressMass=0; %
duvetandSheetsMass=0; %
Sofafabricmass=0; %no sofa

SoftMass=0;

woodPlasticMass=roomArea*35-SoftMass;
woodPlasticMass=roomArea*35-SoftMass;    
    
end





softDensityA=60;
softDensityB=80;
softThicknessA=0.15; %represents thicker furnishings (sofa foam etc.)
softThicknessB=0.01; %Represents thinner funishings (e.g. carpet)

SoftMassA=duvetandSheetsMass+Sofafabricmass+matressMass;
SoftMassB=CurtainMass;

SoftVolumeA=SoftMassA/softDensityA;
SoftVolumeB=SoftMassA/softDensityB;

approxSoftA_SA=(SoftVolumeA/softThicknessA);%no 2* here due to one surface usually being obscured
approxSoftB_SA=(SoftVolumeB/softThicknessB);%as above

Softradius=3*((SoftVolumeA+SoftVolumeB)/(approxSoftA_SA+approxSoftB_SA));
SoftbiotNumber=(10/0.03)*((SoftVolumeA+SoftVolumeB)/(approxSoftA_SA+approxSoftB_SA));% appropriate for typical soft furnishings with conductivity 0.03 w/mK and convective transfer coefficient 10 W/k m2 
SoftFBI=1/(0.282*SoftbiotNumber+0.944);
excessSurfSoft=SoftFBI*excessMeanSoft;
softHeatTransfertoroom=excessSurfSoft*10*(approxSoftA_SA+approxSoftB_SA);
deltaTsoftMean=-softHeatTransfertoroom/(softDensityA*SoftVolumeA*1400+softDensityB*SoftVolumeB*1400);

if isnan(deltaTsoftMean)==1
deltaTsoftMean=0;
else
end
    
woodPlasticDensity=800; %600kg/m^3 as of Influence of internal thermal mass on the indoor thermal dynamics and integration of phase change materials in furniture for building energy storage: A review
woodPlasticThickness=0.018; %0.018m typical as of as of Influence of internal thermal mass on the indoor thermal dynamics and integration of phase change materials in furniture for building energy storage: A review
woodPlasticVolume=woodPlasticMass/woodPlasticDensity;
approxWoodPlasticSA=(woodPlasticVolume/woodPlasticThickness); %a rough surface area calculation for the wooden elements

radius=3*woodPlasticVolume/approxWoodPlasticSA;
biotNumber=(10/0.2)*(woodPlasticVolume/approxWoodPlasticSA);% appropriate for typical wood with conductivity 0.2 w/mK and convective transfer coefficient 10 W/k m2 
FBI=1/(0.282*biotNumber+0.944);
excessSurfWoodPlastic=FBI*excessMeanWoodPlastic;
woodPlasticHeatTransfertoroom=excessSurfWoodPlastic*10*approxWoodPlasticSA;
deltaTWoodPlasticMean=-woodPlasticHeatTransfertoroom/(800*woodPlasticVolume*1700);% heat capacity of wodd and plastic is assumer 1700 J/Kg, they are very close in capacity anyway (1.76 wood, 1.67 plastic)

deltaTWoodPlasticMean(isnan(deltaTWoodPlasticMean))=0;

softHeatTransfertoroom(isnan(softHeatTransfertoroom))=0;

%end
